simulink model "model_3DOF"  (R2022a)
settings: Solver=VariableStepAuto  StartTime=0.0  StopTime=sim_time  RelTol=1e-3
values from neighbouring files (symbols this model uses):
  current_direction = 90*(pi/180)    (= 1.57079632679)    [model_init.m]
  current_speed = 0.0    (= 0)    [model_init.m]
  eta0 = zeros(3,1)    [model_init.m]
  Hs = 3    [model_init.m]
  logging_frequency = 10    [model_init.m]
  nu0 = [1;0;0]    [model_init.m]
  speed_model = [ 0.116392998053662;                 0.214487083945715;                 0.0880678632611925;                -0.00635496887217675;                 0.0937464223577265;                 0.238364678400396]    [model_init.m]
  Tp = 10    [model_init.m]
  wave_dir = 90*(pi/180)    (= 1.57079632679)    [model_init.m]
  wind_direction = 90*(pi/180)    (= 1.57079632679)    [model_init.m]
  wind_speed = 5    [model_init.m]
undefined symbols (not defined in the file or in its folder): vessel
settings Model: Creator=henning  LastModifiedBy=henning

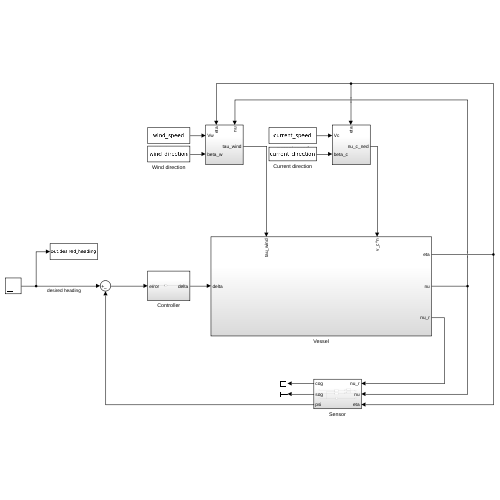
[thumbnail: Simulink's stored preview of the top-level diagram]
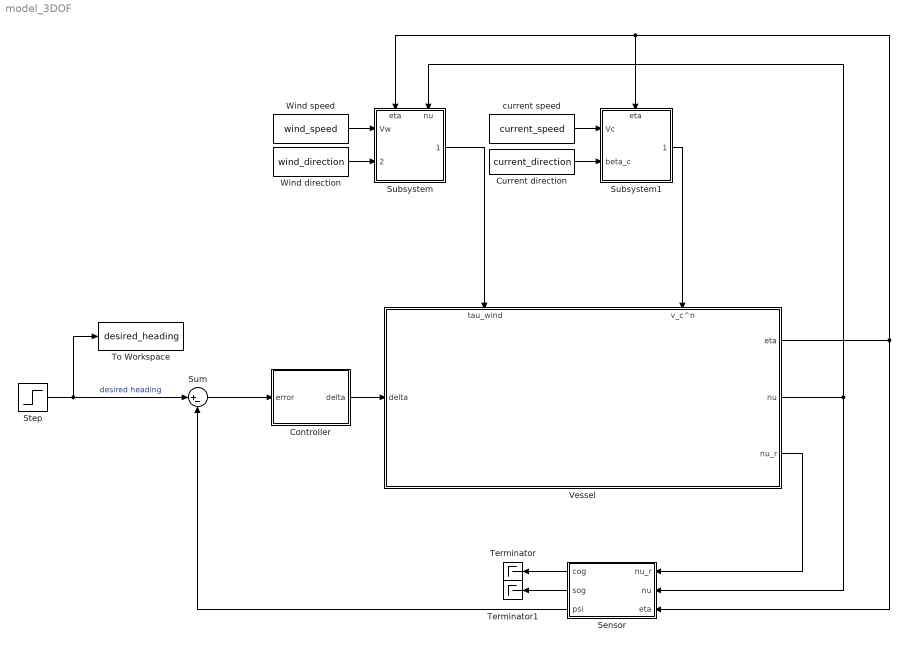
== system model_3DOF ==
  Controller : Subsystem
  Current direction : Constant  Value=current_direction
  Sensor : Subsystem
  Step : Step  Time=10  After=45*(pi/180)  SampleTime=0
  Subsystem : Subsystem
      settings: PortSchema="{\"entries\":[{\"content\":{\"sides\":[{\"content\":{\"connectorIds\":[\"In1\",\"In2\"]},\"type\":\"ConnectorPlacement.EquallySpacedRectSide\",\"uuid\":\"27e31437-fc66-4812-8c01-ad3068482e71\"},{\"content\":{\"connectorIds\":[\"Out1\"],\"side\":\"RIGHT\"},\"type\":\"ConnectorPlacement.EquallySpacedRectSide\",\"uuid\":\"320c9997-0580-44f4-824a-96e160402b2a\"},{\"content\":{\"connectorIds\":[\"In3\",\"In4\"],\"side\":\"TOP\"},\"type\":\"ConnectorPlacement.EquallySpacedRectSide\",\"uuid\":\"c6617624-2adb-4af3-9984-87011c5eff22\"}]},\"type\":\"ConnectorPlacement.EquallySpacedConnector\",\"uuid\":\"8b97342b-acb2-424d-8eeb-6823459b69aa\"}],\"packageUris\":[\"http://schema.mathworks.com/mf0/Connector/R2020b\"],\"version\":\"1.0\"}"
  Subsystem1 : Subsystem
      settings: PortSchema="{\"entries\":[{\"content\":{\"sides\":[{\"content\":{\"connectorIds\":[\"In1\",\"In2\"]},\"type\":\"ConnectorPlacement.EquallySpacedRectSide\",\"uuid\":\"27e31437-fc66-4812-8c01-ad3068482e71\"},{\"content\":{\"connectorIds\":[\"Out1\"],\"side\":\"RIGHT\"},\"type\":\"ConnectorPlacement.EquallySpacedRectSide\",\"uuid\":\"320c9997-0580-44f4-824a-96e160402b2a\"},{\"content\":{\"connectorIds\":[\"In3\"],\"side\":\"TOP\"},\"type\":\"ConnectorPlacement.EquallySpacedRectSide\",\"uuid\":\"c6617624-2adb-4af3-9984-87011c5eff22\"}]},\"type\":\"ConnectorPlacement.EquallySpacedConnector\",\"uuid\":\"8b97342b-acb2-424d-8eeb-6823459b69aa\"}],\"packageUris\":[\"http://schema.mathworks.com/mf0/Connector/R2020b\"],\"version\":\"1.0\"}"
  Sum : Sum  Inputs=|+-
  Terminator : Terminator
  Terminator1 : Terminator
  To Workspace : ToWorkspace  VariableName=desired_heading  SaveFormat=Structure With Time  SampleTime=1/logging_frequency
  Vessel : Subsystem
      settings: PortSchema="{\"entries\":[{\"content\":{\"sides\":[{\"content\":{\"connectorIds\":[\"In1\"]},\"type\":\"ConnectorPlacement.EquallySpacedRectSide\",\"uuid\":\"a9cd8099-9f3b-4f30-b97f-455d882a276b\"},{\"content\":{\"connectorIds\":[\"Out1\",\"Out2\",\"Out3\"],\"side\":\"RIGHT\"},\"type\":\"ConnectorPlacement.EquallySpacedRectSide\",\"uuid\":\"80c625be-d93d-4b24-901e-e53da0ff24c4\"},{\"content\":{\"connectorIds\":[\"In2\",\"In3\"],\"side\":\"TOP\"},\"type\":\"ConnectorPlacement.EquallySpacedRectSide\",\"uuid\":\"f02cbdbd-bc38-407d-9eb9-f7f92cd15c1c\"}]},\"type\":\"ConnectorPlacement.EquallySpacedConnector\",\"uuid\":\"b021f8fe-8c02-464e-8059-ed72840cc3e3\"}],\"packageUris\":[\"http://schema.mathworks.com/mf0/Connector/R2020b\"],\"version\":\"1.0\"}"
  Wind direction : Constant  Value=wind_direction
  Wind speed : Constant  Value=wind_speed
  current speed : Constant  Value=current_speed
  wires:
  Vessel/1(eta) -> Sensor/3(eta), Subsystem1/3(eta), Subsystem/3(eta)
  Vessel/2(nu) -> Sensor/2(nu), Subsystem/4(nu)
  Wind speed/1 -> Subsystem/1(Vw)
  Subsystem/1(tau_wind) -> Vessel/2(tau_wind)
  Wind direction/1 -> Subsystem/2(beta_w)
  Step/1 -> To Workspace/1, Sum/1  "desired heading"
  Sum/1 -> Controller/1(error)
  Controller/1(delta) -> Vessel/1(delta)
  Subsystem1/1(nu_c_ned) -> Vessel/3(v_c^n)
  current speed/1 -> Subsystem1/1(Vc)
  Current direction/1 -> Subsystem1/2(beta_c)
  Sensor/3(psi) -> Sum/2
  Vessel/3(nu_r) -> Sensor/1(nu_r)
  Sensor/1(cog) -> Terminator/1
  Sensor/2(sog) -> Terminator1/1

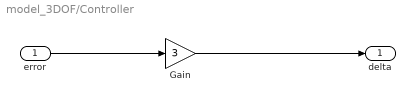
== system model_3DOF/Controller ==
  error : Inport
  Gain : Gain  Gain=3
  delta : Outport
  wires:
  Gain/1 -> delta/1
  error/1 -> Gain/1

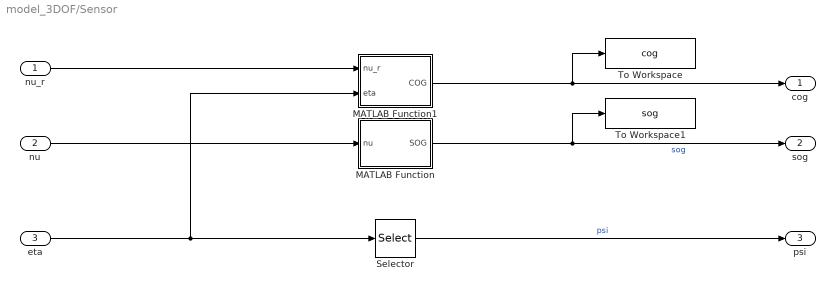
== system model_3DOF/Sensor ==
  nu_r : Inport
  nu : Inport  Port=2
  eta : Inport  Port=3
  MATLAB Function : MATLAB Function  TreatAsAtomicUnit=on
  MATLAB Function1 : MATLAB Function  TreatAsAtomicUnit=on
  Selector : Selector  InputPortWidth=3  IndexOptions=Index vector (dialog)  Indices=[3]  OutputSizes=1
  To Workspace : ToWorkspace  VariableName=cog  SaveFormat=Structure With Time  SampleTime=1/logging_frequency
  To Workspace1 : ToWorkspace  VariableName=sog  SaveFormat=Structure With Time  SampleTime=1/logging_frequency
  cog : Outport
  sog : Outport  Port=2
  psi : Outport  Port=3
  wires:
  eta/1 -> MATLAB Function1/2(eta), Selector/1
  Selector/1 -> psi/1  "psi"
  nu/1 -> MATLAB Function/1(nu)
  MATLAB Function/1(SOG) -> To Workspace1/1, sog/1  "sog"
  nu_r/1 -> MATLAB Function1/1(nu_r)
  MATLAB Function1/1(COG) -> To Workspace/1, cog/1

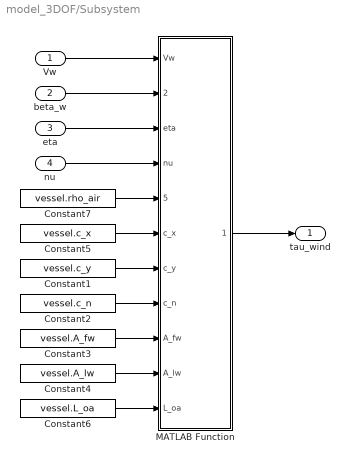
== system model_3DOF/Subsystem ==
  Vw : Inport
  beta_w : Inport  Port=2
  eta : Inport  Port=3
  nu : Inport  Port=4
  Constant1 : Constant  Value=vessel.c_y
  Constant2 : Constant  Value=vessel.c_n
  Constant3 : Constant  Value=vessel.A_fw
  Constant4 : Constant  Value=vessel.A_lw
  Constant5 : Constant  Value=vessel.c_x
  Constant6 : Constant  Value=vessel.L_oa
  Constant7 : Constant  Value=vessel.rho_air
  MATLAB Function : MATLAB Function  TreatAsAtomicUnit=on
  tau_wind : Outport
  wires:
  Vw/1 -> MATLAB Function/1(Vw)
  MATLAB Function/1(tau_wind) -> tau_wind/1
  beta_w/1 -> MATLAB Function/2(beta_w)
  Constant5/1 -> MATLAB Function/6(c_x)
  Constant1/1 -> MATLAB Function/7(c_y)
  Constant2/1 -> MATLAB Function/8(c_n)
  Constant3/1 -> MATLAB Function/9(A_fw)
  Constant4/1 -> MATLAB Function/10(A_lw)
  Constant6/1 -> MATLAB Function/11(L_oa)
  Constant7/1 -> MATLAB Function/5(rho_air)
  eta/1 -> MATLAB Function/3(eta)
  nu/1 -> MATLAB Function/4(nu)

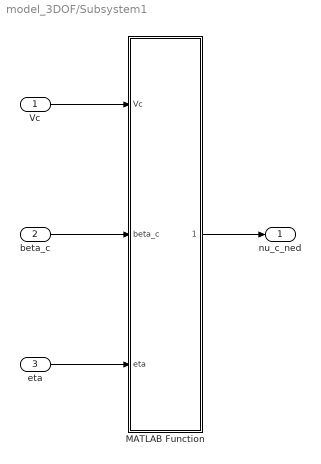
== system model_3DOF/Subsystem1 ==
  Vc : Inport
  beta_c : Inport  Port=2
  eta : Inport  Port=3
  MATLAB Function : MATLAB Function  TreatAsAtomicUnit=on
  nu_c_ned : Outport
  wires:
  Vc/1 -> MATLAB Function/1(Vc)
  MATLAB Function/1(u_c_ned) -> nu_c_ned/1
  beta_c/1 -> MATLAB Function/2(beta_c)
  eta/1 -> MATLAB Function/3(eta)

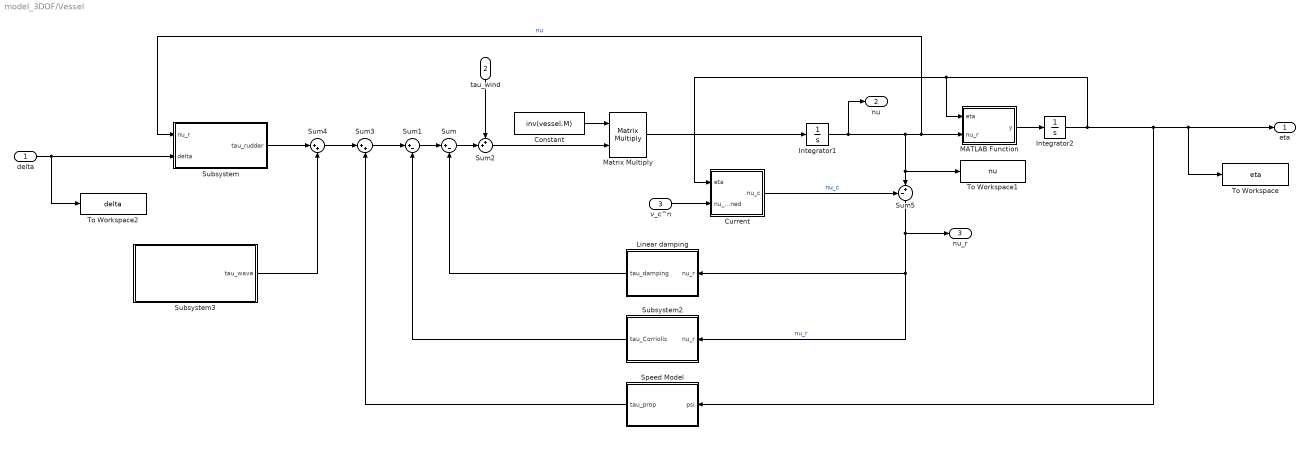
== system model_3DOF/Vessel ==
  delta : Inport
  tau_wind : Inport  Port=2
  v_c^n : Inport  Port=3
  Constant : Constant  Value=inv(vessel.M)
  Current : Subsystem
  Integrator1 : Integrator  InitialCondition=nu0
  Integrator2 : Integrator  InitialCondition=eta0
  Linear damping : Subsystem
  MATLAB Function : MATLAB Function  TreatAsAtomicUnit=on
  Matrix Multiply : Product  Multiplication=Matrix(*)
  Speed Model : Subsystem
  Subsystem : Subsystem
  Subsystem2 : Subsystem
  Subsystem3 : Subsystem
  Sum : Sum  Inputs=|+-
  Sum1 : Sum  Inputs=|+-
  Sum2 : Sum  Inputs=++|
  Sum3 : Sum  Inputs=|++
  Sum4 : Sum  Inputs=|++
  Sum5 : Sum  Inputs=-+|
  To Workspace : ToWorkspace  VariableName=eta  SaveFormat=Structure With Time  SampleTime=1/logging_frequency
  To Workspace1 : ToWorkspace  VariableName=nu  SaveFormat=Structure With Time  SampleTime=1/logging_frequency
  To Workspace2 : ToWorkspace  VariableName=delta  SaveFormat=Structure With Time  SampleTime=1/logging_frequency
  eta : Outport
  nu : Outport  Port=2
  nu_r : Outport  Port=3
  wires:
  Matrix Multiply/1 -> Integrator1/1
  Linear damping/1(tau_damping) -> Sum/2
  Subsystem2/1(tau_Corriolis) -> Sum1/2
  Sum1/1 -> Sum/1
  Integrator1/1 -> nu/1, MATLAB Function/2(nu_r), Subsystem/1(nu_r), To Workspace1/1, Sum5/2  "nu"
  MATLAB Function/1(y) -> Integrator2/1
  Constant/1 -> Matrix Multiply/1
  delta/1 -> To Workspace2/1, Subsystem/2(delta)
  Sum2/1 -> Matrix Multiply/2
  Sum/1 -> Sum2/2
  Integrator2/1 -> Speed Model/1(psi), To Workspace/1, eta/1, Current/1(eta), MATLAB Function/1(eta)
  Sum3/1 -> Sum1/1
  tau_wind/1 -> Sum2/1
  Speed Model/1(tau_prop) -> Sum3/2
  Subsystem/1(tau_rudder) -> Sum4/1
  Sum4/1 -> Sum3/1
  Sum5/1 -> nu_r/1, Subsystem2/1(nu_r), Linear damping/1(nu_r)  "nu_r"
  v_c^n/1 -> Current/2(nu_c_ned)
  Current/1(nu_c) -> Sum5/1  "nu_c"
  Subsystem3/1(tau_wave) -> Sum4/2

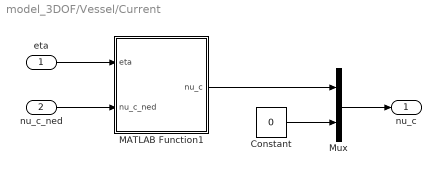
== system model_3DOF/Vessel/Current ==
  eta : Inport
  nu_c_ned : Inport  Port=2
  Constant : Constant  Value=0
  MATLAB Function1 : MATLAB Function  TreatAsAtomicUnit=on
  Mux : Mux  Inputs=2
  nu_c : Outport
  wires:
  nu_c_ned/1 -> MATLAB Function1/2(nu_c_ned)
  eta/1 -> MATLAB Function1/1(eta)
  MATLAB Function1/1(nu_c) -> Mux/1
  Mux/1 -> nu_c/1
  Constant/1 -> Mux/2

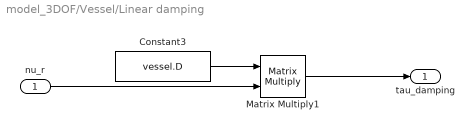
== system model_3DOF/Vessel/Linear damping ==
  nu_r : Inport
  Constant3 : Constant  Value=vessel.D
  Matrix Multiply1 : Product  Multiplication=Matrix(*)
  tau_damping : Outport
  wires:
  Matrix Multiply1/1 -> tau_damping/1
  Constant3/1 -> Matrix Multiply1/1
  nu_r/1 -> Matrix Multiply1/2

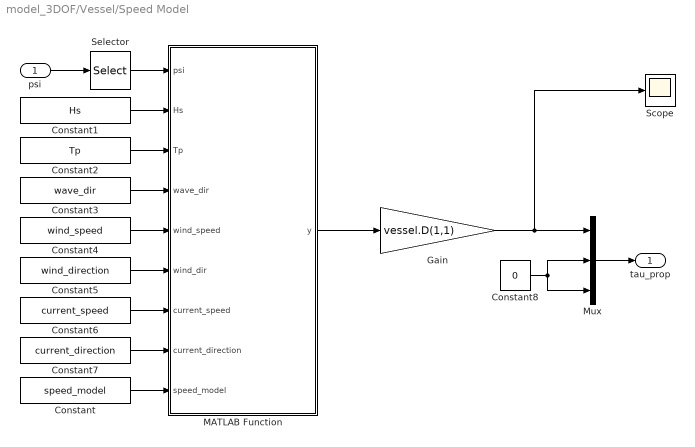
== system model_3DOF/Vessel/Speed Model ==
  psi : Inport
  Constant : Constant  Value=speed_model
  Constant1 : Constant  Value=Hs
  Constant2 : Constant  Value=Tp
  Constant3 : Constant  Value=wave_dir
  Constant4 : Constant  Value=wind_speed
  Constant5 : Constant  Value=wind_direction
  Constant6 : Constant  Value=current_speed
  Constant7 : Constant  Value=current_direction
  Constant8 : Constant  Value=0
  Gain : Gain  Gain=vessel.D(1,1)
  MATLAB Function : MATLAB Function  TreatAsAtomicUnit=on
  Mux : Mux  Inputs=3
  Scope : Scope
  Selector : Selector  InputPortWidth=3  IndexOptions=Index vector (dialog)  Indices=[3]  OutputSizes=1
  tau_prop : Outport
  wires:
  MATLAB Function/1(y) -> Gain/1
  Constant/1 -> MATLAB Function/9(speed_model)
  Constant1/1 -> MATLAB Function/2(Hs)
  Constant2/1 -> MATLAB Function/3(Tp)
  Constant3/1 -> MATLAB Function/4(wave_dir)
  Constant4/1 -> MATLAB Function/5(wind_speed)
  Constant5/1 -> MATLAB Function/6(wind_dir)
  Constant6/1 -> MATLAB Function/7(current_speed)
  Constant7/1 -> MATLAB Function/8(current_direction)
  psi/1 -> Selector/1
  Selector/1 -> MATLAB Function/1(psi)
  Gain/1 -> Scope/1, Mux/1
  Constant8/1 -> Mux/2, Mux/3
  Mux/1 -> tau_prop/1

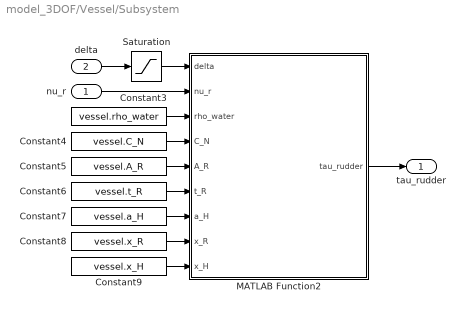
== system model_3DOF/Vessel/Subsystem ==
  nu_r : Inport
  delta : Inport  Port=2
  Constant3 : Constant  Value=vessel.rho_water
  Constant4 : Constant  Value=vessel.C_N
  Constant5 : Constant  Value=vessel.A_R
  Constant6 : Constant  Value=vessel.t_R
  Constant7 : Constant  Value=vessel.a_H
  Constant8 : Constant  Value=vessel.x_R
  Constant9 : Constant  Value=vessel.x_H
  MATLAB Function2 : MATLAB Function  TreatAsAtomicUnit=on
  Saturation : Saturate  UpperLimit=vessel.rudder_saturation  LowerLimit=-vessel.rudder_saturation
  tau_rudder : Outport
  wires:
  Constant3/1 -> MATLAB Function2/3(rho_water)
  Constant4/1 -> MATLAB Function2/4(C_N)
  Constant5/1 -> MATLAB Function2/5(A_R)
  Constant6/1 -> MATLAB Function2/6(t_R)
  Constant7/1 -> MATLAB Function2/7(a_H)
  Constant8/1 -> MATLAB Function2/8(x_R)
  Constant9/1 -> MATLAB Function2/9(x_H)
  delta/1 -> Saturation/1
  nu_r/1 -> MATLAB Function2/2(nu_r)
  MATLAB Function2/1(tau_rudder) -> tau_rudder/1
  Saturation/1 -> MATLAB Function2/1(delta)

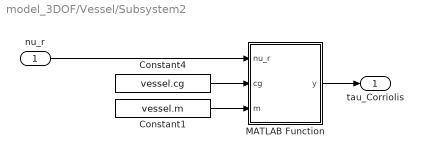
== system model_3DOF/Vessel/Subsystem2 ==
  nu_r : Inport
  Constant1 : Constant  Value=vessel.m
  Constant4 : Constant  Value=vessel.cg
  MATLAB Function : MATLAB Function  TreatAsAtomicUnit=on
  tau_Corriolis : Outport
  wires:
  nu_r/1 -> MATLAB Function/1(nu_r)
  Constant4/1 -> MATLAB Function/2(cg)
  Constant1/1 -> MATLAB Function/3(m)
  MATLAB Function/1(y) -> tau_Corriolis/1

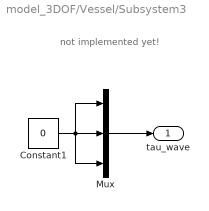
== system model_3DOF/Vessel/Subsystem3 ==
  note: not implemented yet!
  Constant1 : Constant  Value=0
  Mux : Mux  Inputs=3
  tau_wave : Outport
  wires:
  Constant1/1 -> Mux/3, Mux/1, Mux/2
  Mux/1 -> tau_wave/1

== matlab function model_3DOF/Sensor/MATLAB Function ==
  data: nu input; SOG output
function SOG = fcn(nu)

SOG = sqrt(nu(1)^2 + nu(2)^2);

== matlab function model_3DOF/Sensor/MATLAB Function1 ==
  data: nu_r input; COG output; eta input
function COG = fcn(nu_r, eta)
psi = eta(3);
Ur = sqrt(nu_r(1)^2 + nu_r(2)^2);
beta = asin(nu_r(2) / Ur);
COG = psi + beta;

== matlab function model_3DOF/Vessel/Subsystem2/MATLAB Function ==
  data: nu_r input; y output; cg input; m input
function y = fcn(nu_r,cg, m)
    r = nu_r(3);
    C = [0        -m*r -m*cg(1)*r;...
         m*r         0      0     ;...
         m*cg(1)*r  0      0     ];
y = C*nu_r;

== matlab function model_3DOF/Subsystem/MATLAB Function ==
  data: Vw input; beta_w input; tau_wind output; eta input; nu input; rho_air input; c_x input; c_y input; c_n input; A_fw input; A_lw input; L_oa input
function tau_wind = fcn(Vw, beta_w, eta, nu, rho_air, c_x, c_y, c_n, A_fw, A_lw, L_oa)
psi = eta(3);
u = nu(1);
v = nu(2);
u_w = Vw*cos(beta_w - psi);
v_w = Vw*sin(beta_w - psi);
u_rw = u - u_w;
v_rw = v - v_w;

Vrw = sqrt(u_rw^2 + v_rw^2);
gamma = -atan2(v_rw,u_rw);
q = 0.5*rho_air*Vrw^2;
tau_wind = [-c_x*cos(gamma)*q*A_fw;...
             c_y*sin(gamma)*q*A_lw;...
             c_n*sin(2*gamma)*q*A_lw*L_oa];

== matlab function model_3DOF/Vessel/MATLAB Function ==
  data: eta input; nu_r input; y output
function y = fcn(eta, nu_r)
    psi = eta(3);
    R = [cos(psi) -sin(psi) 0;...
         sin(psi)  cos(psi) 0;...
            0         0     1];
y = R*nu_r;

== matlab function model_3DOF/Vessel/Subsystem/MATLAB Function2 ==
  data: delta input; nu_r input; tau_rudder output; rho_water input; C_N input; A_R input; t_R input; a_H input; x_R input; x_H input
function tau_rudder = rudder_force(delta, nu_r, rho_water, C_N, A_R, t_R, a_H, x_R, x_H)


% Relative speed
Ur = sqrt(nu_r(1)^2+nu_r(2)^2);

% Effective Rudder angle
alphar = delta - atan(nu_r(2)/nu_r(1));

% Rudder normal force
F_normal = 0.5*rho_water*Ur^2*C_N*A_R*sin(alphar);


% Rudder forces in 3-DOF
tau_rudder = [-(1-t_R)*F_normal*sin(delta);...
             -(1+a_H)*F_normal*cos(delta);...
             -(x_R + a_H*x_H)*F_normal*cos(delta)];

== matlab function model_3DOF/Vessel/Speed Model/MATLAB Function ==
  data: psi input; Hs input; Tp input; wave_dir input; y output; wind_speed input; wind_dir input; current_speed input; current_direction input; speed_model input
function y = fcn(psi, Hs, Tp, wave_dir, wind_speed, wind_dir, current_speed, current_direction, speed_model)
 feature_vector = [Hs;...
                   (2*pi)/Tp;...
                   cos(wave_dir);... % Pi or not?
                   wind_speed*cos(psi - wind_dir - pi);...
                   current_speed*cos(current_direction);...
                   1];
y = feature_vector' * speed_model;

== matlab function model_3DOF/Vessel/Current/MATLAB Function1 ==
  data: eta input; nu_c_ned input; nu_c output
function nu_c = fcn(eta, nu_c_ned)
    psi = eta(3);
    R = [cos(psi) -sin(psi);...
         sin(psi)  cos(psi)];
nu_c = R'*nu_c_ned;

== matlab function model_3DOF/Subsystem1/MATLAB Function ==
  data: Vc input; beta_c input; u_c_ned output; eta input
function u_c_ned = fcn(Vc, beta_c, eta)
psi = eta(3);

u_c_north = Vc*cos(beta_c - psi);
u_c_east  = Vc*sin(beta_c - psi);

u_c_ned = [u_c_north;...
           u_c_east];
